simulink model "Vehiculo"  (R2020a)
settings: Solver=VariableStepAuto  StartTime=0.0  StopTime=180  RelTol=1e-3
PreLoadFcn:
  | Parametros_vehiculo
values from neighbouring files (symbols this model uses):
  fr = 0.8    [Parametros_vehiculo.m]
  g = 9.81    [Parametros_vehiculo.m]
  inclinacion = deg2rad(15)    [Parametros_vehiculo.m]
  K_drag = 0.5 * rho_aire * C_d * A_f    (= 0.590625)    [Parametros_vehiculo.m]
  M = 600    [Parametros_vehiculo.m]
  r_rueda = 0.3    [Parametros_vehiculo.m]
undefined symbols (not defined in the file or in its folder): T0, Tf, v0
settings Model: Creator=pablo  LastModifiedBy=pablo

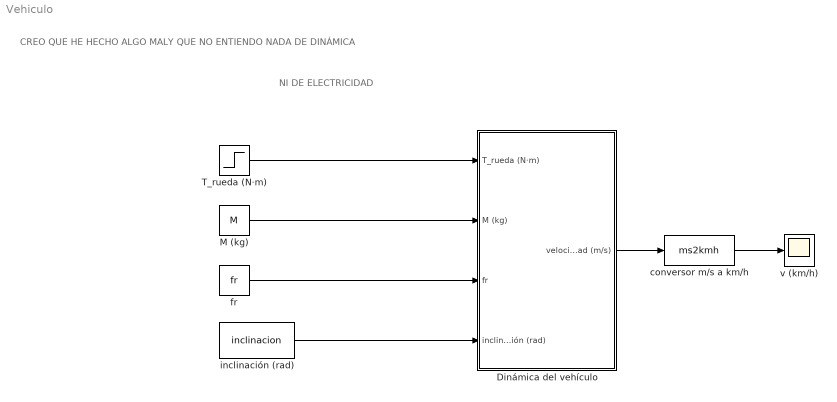
== system Vehiculo ==
  note: NI DE ELECTRICIDAD
  note: CREO QUE HE HECHO ALGO MALY QUE NO ENTIENDO NADA DE DINÁMICA
  Dinámica del vehículo : Subsystem
  M (kg) : Constant  Value=M
  T_rueda (N·m) : Step  Time=10  Before=T0  After=Tf  SampleTime=0
  conversor m/s a km/h : MATLABFcn  MATLABFcn=ms2kmh  OutputDimensions=1
  fr : Constant  Value=fr
  inclinación (rad) : Constant  Value=inclinacion
  v (km/h) : Scope
  wires:
  Dinámica del vehículo/1(velocidad (m/s)) -> conversor m/s a km/h/1
  fr/1 -> Dinámica del vehículo/3(fr)
  inclinación (rad)/1 -> Dinámica del vehículo/4(inclinación (rad))
  M (kg)/1 -> Dinámica del vehículo/2(M (kg))
  T_rueda (N·m)/1 -> Dinámica del vehículo/1(T_rueda (N·m))
  conversor m/s a km/h/1 -> v (km/h)/1

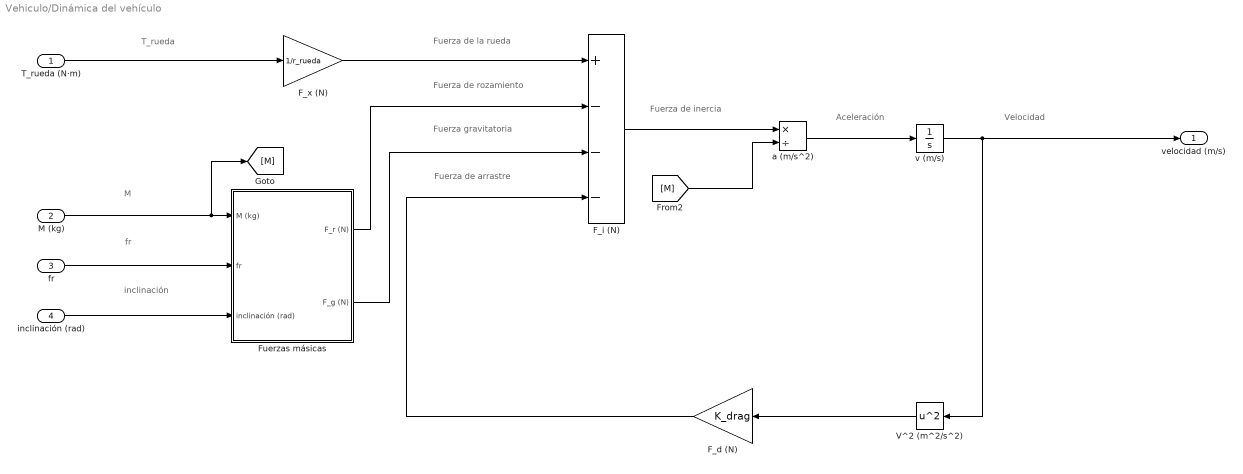
== system Vehiculo/Dinámica del vehículo ==
  note: fr
  note: inclinación
  note: M
  note: Fuerza gravitatoria
  note: Fuerza de rozamiento
  note: Fuerza de la rueda
  note: Fuerza de inercia
  note: Aceleración
  note: Velocidad
  note: Fuerza de arrastre
  note: T_rueda
  T_rueda (N·m) : Inport
  M (kg) : Inport  Port=2
  fr : Inport  Port=3
  inclinación (rad) : Inport  Port=4
  F_d (N) : Gain  Gain=K_drag
  F_i (N) : Sum  Inputs=+---
  F_x (N) : Gain  Gain=1/r_rueda
  Fuerzas másicas : Subsystem
  V^2 (m^2/s^2) : Math  Operator=square  SaturateOnIntegerOverflow=on
  a (m/s^2) : Product  Inputs=*/
  v (m/s) : Integrator  InitialCondition=v0
  velocidad (m/s) : Outport
  wires:
  [M] -> a (m/s^2)/2
  a (m/s^2)/1 -> v (m/s)/1
  V^2 (m^2/s^2)/1 -> F_d (N)/1
  Fuerzas másicas/2(F_g (N)) -> F_i (N)/3
  M (kg)/1 -> [M], Fuerzas másicas/1(M (kg))
  F_x (N)/1 -> F_i (N)/1
  F_d (N)/1 -> F_i (N)/4
  Fuerzas másicas/1(F_r (N)) -> F_i (N)/2
  F_i (N)/1 -> a (m/s^2)/1
  v (m/s)/1 -> V^2 (m^2/s^2)/1, velocidad (m/s)/1
  fr/1 -> Fuerzas másicas/2(fr)
  inclinación (rad)/1 -> Fuerzas másicas/3(inclinación (rad))
  T_rueda (N·m)/1 -> F_x (N)/1

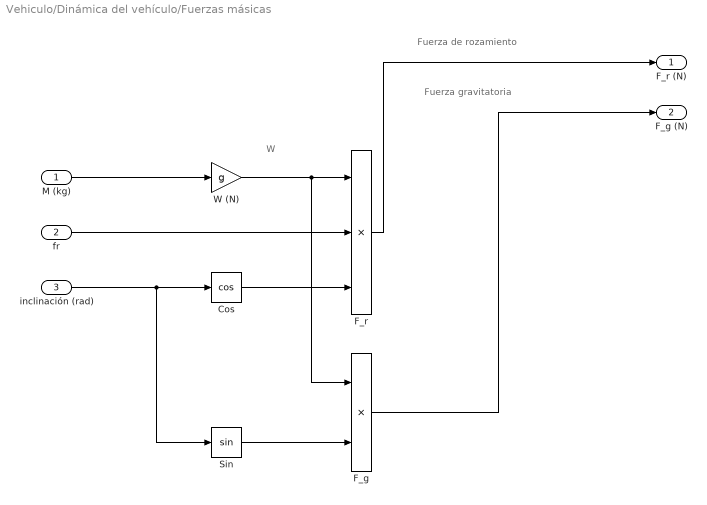
== system Vehiculo/Dinámica del vehículo/Fuerzas másicas ==
  note: Fuerza gravitatoria
  note: Fuerza de rozamiento
  note: W
  M (kg) : Inport
  fr : Inport  Port=2
  inclinación (rad) : Inport  Port=3
  Cos : Trigonometry  Operator=cos
  F_g : Product
  F_r : Product  Inputs=3
  Sin : Trigonometry
  W (N) : Gain  Gain=g
  F_r (N) : Outport
  F_g (N) : Outport  Port=2
  wires:
  fr/1 -> F_r/2
  inclinación (rad)/1 -> Sin/1, Cos/1
  F_g/1 -> F_g (N)/1
  W (N)/1 -> F_g/1, F_r/1
  Cos/1 -> F_r/3
  Sin/1 -> F_g/2
  F_r/1 -> F_r (N)/1
  M (kg)/1 -> W (N)/1
